simulink model "SImple"  (Simulink 7.9)
settings: Solver=ode45  StartTime=0.0  StopTime=t  MaxStep=0.001  RelTol=1e-3
values from neighbouring files (symbols this model uses):
  beta = 0.7    [SEIR.m]    (also in SI.m = 0.1; SIR.m = 0.4; modele_epidemiologiczne.m = str2num(get(handles.edit6, 'String')))
  I0 = str2num(get(handles.edit3, 'String'))    [modele_epidemiologiczne.m]
settings Model: Creator=Olka  LastModifiedBy=Zaneta
settings SolverCC: AutoInsertRateTranBlk=on
settings DataIOCC: LimitDataPoints=off  SaveCompleteFinalSimState=on
settings DebuggingCC: FcnCallInpInsideContextMsg=Use local settings
settings GRTTargetCC: CombineOutputUpdateFcns=off  GRTInterface=on

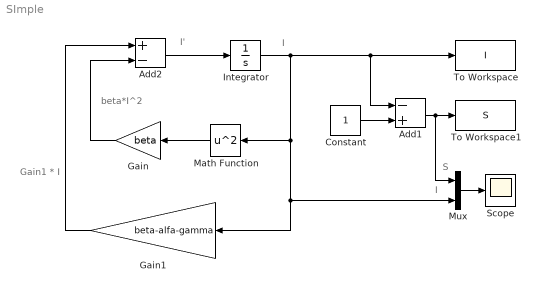
== system SImple ==
  note: I'
  note: I
  note: beta*I^2
  note: Gain1 * I
  note: S
  note: I
  Add1 : Sum  Inputs=-+
  Add2 : Sum  Inputs=+-
  Constant : Constant
  Gain : Gain  Gain=beta
  Gain1 : Gain  Gain=beta-alfa-gamma
  Integrator : Integrator  InitialCondition=I0
  Math Function : Math  Operator=square  SaturateOnIntegerOverflow=on
  Mux : Mux  Inputs=2
  Scope : Scope
      settings: TimeRange=20  YMin=0.35  YMax=0.7000000000000001
  To Workspace : ToWorkspace  VariableName=I  SampleTime=-1
  To Workspace1 : ToWorkspace  VariableName=S  SampleTime=-1
  wires:
  Integrator/1 -> Add1/1, To Workspace/1, Math Function/1, Gain1/1, Mux/2
  Math Function/1 -> Gain/1
  Gain/1 -> Add2/2
  Gain1/1 -> Add2/1
  Constant/1 -> Add1/2
  Add1/1 -> To Workspace1/1, Mux/1
  Add2/1 -> Integrator/1
  Mux/1 -> Scope/1
